simulink model "dirt_deriv_test_BAG"  (R2014b)
settings: Solver=ode45  StartTime=0.0  StopTime=3  RelTol=1e-3
values from neighbouring files (symbols this model uses):
  A = diag(a_sup_diag,1)    [num_der.m]    (also in num_der_poly.m; num_der_trig.m)
  B = [zeros(M-2,1);1]    [num_der.m]    (also in num_der_poly.m; num_der_trig.m)
  C = Coeff(:,[1:1:M-1])    [num_der.m]    (also in num_der_poly.m; num_der_trig.m)
  D = Coeff(:,M)    [num_der.m]    (also in num_der_poly.m; num_der_trig.m)
  M = 20,m0=10, Dt=.0005, W=[1:1:3]*pi/(M*Dt),Q=diag([1:1:M])    [num_deriv_trig_design.m]
undefined symbols (not defined in the file or in its folder): Dt
libraries: simulink x1
settings Model: Creator=grizzle  LastModifiedBy=grizzle
settings DataIOCC: LimitDataPoints=off  SignalLoggingSaveFormat=ModelDataLogs  SaveTime=off  TimeSaveName=t
settings OptimizationCC: BooleanDataType=off  ExpressionDepthLimit=2147483647  InitFltsAndDblsToZero=on
settings DebuggingCC: SaveWithParameterizedLinksMsg=none  UnderspecifiedInitializationDetection=Classic  MergeDetectMultiDrivingBlocksExec=none  SignalResolutionControl=TryResolveAllWithWarning  SolverPrmCheckMsg=none  MultiTaskDSMMsg=warning  MultiTaskCondExecSysMsg=none  FcnCallInpInsideContextMsg=UseLocalSettings  StateNameClashWarn=warning  StrictBusMsg=None
settings HardwareCC: TargetUnknown=on
settings RTWCC: IncludeERTFirstTime=on
settings GRTTargetCC: CombineOutputUpdateFcns=off  GRTInterface=on

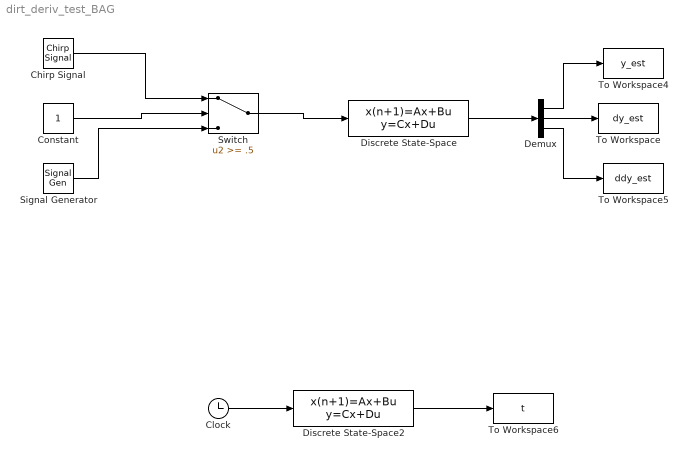
== system dirt_deriv_test_BAG ==
  Chirp Signal : simulink/Sources/Chirp Signal  f1=1  T=5  f2=8
  Clock : Clock
  Constant : Constant
  Demux : Demux  Outputs=3
  Discrete State-Space : DiscreteStateSpace  A=A  B=B  C=C  D=D  X0=zeros(M-1,1);  SampleTime=Dt
  Discrete State-Space2 : DiscreteStateSpace  A=[]  B=[]  C=[]  X0=[]  SampleTime=Dt
  Signal Generator : SignalGenerator  Frequency=3^.5
  Switch : Switch  Threshold=.5
  To Workspace : ToWorkspace  VariableName=dy_est  SampleTime=-1
  To Workspace4 : ToWorkspace  VariableName=y_est  SampleTime=-1
  To Workspace5 : ToWorkspace  VariableName=ddy_est  SampleTime=-1
  To Workspace6 : ToWorkspace  VariableName=t  SampleTime=-1
  wires:
  Discrete State-Space/1 -> Demux/1
  Demux/2 -> To Workspace/1
  Demux/1 -> To Workspace4/1
  Demux/3 -> To Workspace5/1
  Clock/1 -> Discrete State-Space2/1
  Discrete State-Space2/1 -> To Workspace6/1
  Chirp Signal/1 -> Switch/1
  Signal Generator/1 -> Switch/3
  Constant/1 -> Switch/2
  Switch/1 -> Discrete State-Space/1
